simulink model "SuperCtrlStateMachineTest2"  (R2012b)
settings: Solver=ode1  StartTime=0.0  StopTime=Inf  FixedStep=0.001  RelTol=1e-3
PostLoadFcn:
  | , if any(exist('dsrtsu_mdlpostloadfcn', 'file') == [2, 3, 6]), try dsrtsu_mdlpostloadfcn('Execute', bdroot); catch fprintf('Error in PostLoadFcn (dsrtsu_mdlpostloadfcn) for model "%s":\n %s\n', bdroot, lasterr); end, end,
settings Model: DSRTSU_INTERNAL_RTI_VER=430  DSRTSU_INTERNAL_RTI_TYPE=rti1103  DSRTSU_INTERNAL_RTIFPGA=20  BufferReuse=off  Creator=Raghav  LastModifiedBy=Raghav
settings OptimizationCC: BlockReduction=off  OptimizeBlockIOStorage=off  BufferReuse=off  ExpressionFolding=off  LocalBlockOutputs=off
settings HardwareCC: ProdIntDivRoundTo=Zero  ProdEndianess=BigEndian  ProdHWDeviceType=Generic->Custom  TargetIntDivRoundTo=Zero  TargetEndianess=BigEndian  TargetHWDeviceType=Generic->Custom
settings RTWCC: SystemTargetFile=rti1103.tlc  MakeCommand=make_rti  TemplateMakefile=rti1103.tmf  Description=dSPACE DS1103 Hardware Platform  ProcessScript=rti1103_make_rtw_hook
settings STFCustomTargetCC: CodeReplacementLibrary=ANSI_C  ParMdlRefBuildCompliant=on  GeneratePreprocessorConditionals=Disable all  MatFileLogging=on  SystemTargetFile=rti1103.tlc
settings GRTTargetCC: CompOptLevelCompliant=off  ConcurrentExecutionCompliant=off  CombineOutputUpdateFcns=off  GRTInterface=on  ExtModeMexFile=noextcomm

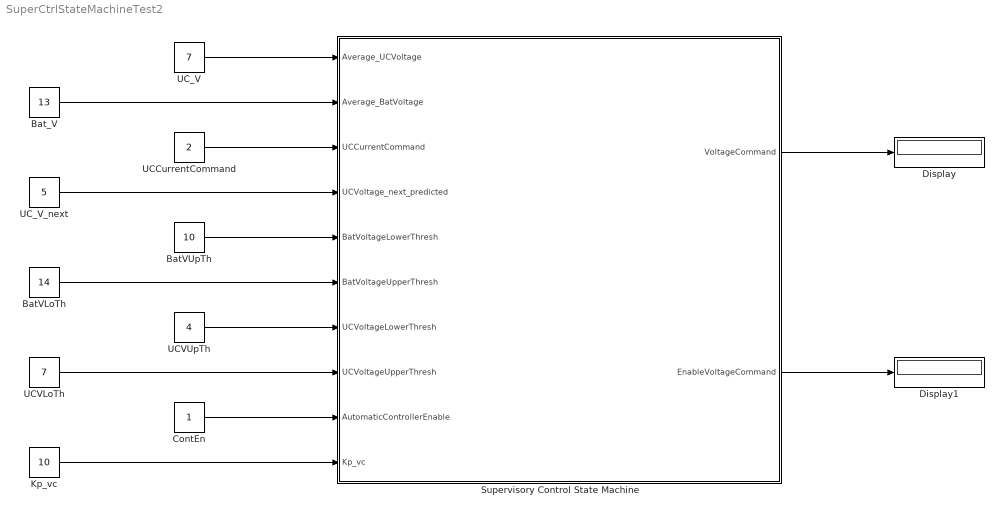
== system SuperCtrlStateMachineTest2 ==
  BatVLoTh : Constant  Value=14
  BatVUpTh : Constant  Value=10
  Bat_V : Constant  Value=13
  ContEn : Constant
  Display : Display
  Display1 : Display
  Kp_vc : Constant  Value=10
  Supervisory Control State Machine : Stateflow chart  TreatAsAtomicUnit=on
  UCCurrentCommand : Constant  Value=2
  UCVLoTh : Constant  Value=7
  UCVUpTh : Constant  Value=4
  UC_V : Constant  Value=7
  UC_V_next : Constant  Value=5
  wires:
  UC_V/1 -> Supervisory Control State Machine/1(Average_UCVoltage)
  Bat_V/1 -> Supervisory Control State Machine/2(Average_BatVoltage)
  UCCurrentCommand/1 -> Supervisory Control State Machine/3(UCCurrentCommand)
  UC_V_next/1 -> Supervisory Control State Machine/4(UCVoltage_next_predicted)
  BatVUpTh/1 -> Supervisory Control State Machine/5(BatVoltageLowerThresh)
  BatVLoTh/1 -> Supervisory Control State Machine/6(BatVoltageUpperThresh)
  UCVUpTh/1 -> Supervisory Control State Machine/7(UCVoltageLowerThresh)
  UCVLoTh/1 -> Supervisory Control State Machine/8(UCVoltageUpperThresh)
  ContEn/1 -> Supervisory Control State Machine/9(AutomaticControllerEnable)
  Kp_vc/1 -> Supervisory Control State Machine/10(Kp_vc)
  Supervisory Control State Machine/1(VoltageCommand) -> Display/1
  Supervisory Control State Machine/2(EnableVoltageCommand) -> Display1/1

== stateflow chart SuperCtrlStateMachineTest2/Supervisory Control State Machine ==
  state InitState
    entry:
    delta_Voltage = 0.1
    VoltageCommand = Average_UCVoltage
    EnableVoltageCommand = 0
  state ChargeDownState
    during:
    VoltageCommand = UCVoltageUpperThresh - delta_Voltage
    EnableVoltageCommand = 1
  state CurrentControlState
    during:
    EnableVoltageCommand = 0
  state ChargeUpState
    during:
    VoltageCommand = UCVoltageLowerThresh + delta_Voltage
    EnableVoltageCommand = 1
  (default) -> InitState
  InitState -> ChargeDownState [order 2] : [( Average_UCVoltage >= UCVoltageUpperThresh ...
      | || Average_BatVoltage <= BatVoltageLowerThresh)...
      | && AutomaticControllerEnable == 1]
  InitState -> ChargeUpState [order 1] : [( Average_UCVoltage <= UCVoltageLowerThresh ...
      | || Average_BatVoltage >= BatVoltageUpperThresh)...
      | && AutomaticControllerEnable == 1]
  ChargeUpState -> InitState [order 2] : [AutomaticControllerEnable==0]
  ChargeDownState -> InitState [order 2] : [AutomaticControllerEnable==0]
  CurrentControlState -> InitState [order 3] : [AutomaticControllerEnable==0]
  InitState -> CurrentControlState [order 3] : [(Average_UCVoltage < UCVoltageUpperThresh ...
      | && Average_UCVoltage > UCVoltageLowerThresh ...
      | && Average_BatVoltage > BatVoltageLowerThresh ...
      | && Average_BatVoltage < BatVoltageUpperThresh)...
      | && AutomaticControllerEnable==1]
  CurrentControlState -> ChargeDownState [order 1] : [ (Average_UCVoltage >= UCVoltageUpperThresh ...
      | || (UCVoltageUpperThresh - UCVoltage_next_predicted)*Kp_vc - UCCurrentCommand < 1 ...
      | || Average_BatVoltage <= BatVoltageLowerThresh) ...
      | && UCCurrentCommand >= 0]
  ChargeDownState -> CurrentControlState [order 1] : [UCCurrentCommand < 0]
  CurrentControlState -> ChargeUpState [order 2] : [ (Average_UCVoltage <= UCVoltageLowerThresh ...
      | || (UCVoltageLowerThresh - UCVoltage_next_predicted)*Kp_vc - UCCurrentCommand > 1 ...
      | || Average_BatVoltage >= BatVoltageUpperThresh) ...
      | && UCCurrentCommand <= 0]
  ChargeUpState -> CurrentControlState [order 1] : [UCCurrentCommand > 0]
  data: Average_UCVoltage input; Average_BatVoltage input; UCCurrentCommand input; UCVoltage_next_predicted input; VoltageCommand output double; EnableVoltageCommand output double; BatVoltageLowerThresh input double; BatVoltageUpperThresh input double; UCVoltageLowerThresh input double; UCVoltageUpperThresh input double; delta_Voltage local double; AutomaticControllerEnable input; Kp_vc input
